simulink model "SAS_12th_question"  (R2024b)
settings: Solver=ode45  StartTime=0.0  StopTime=10.0  RelTol=1e-3
settings Model: Creator=anand  LastModifiedBy=Acer
settings RTWCC: GPUComputeCapability=3.5

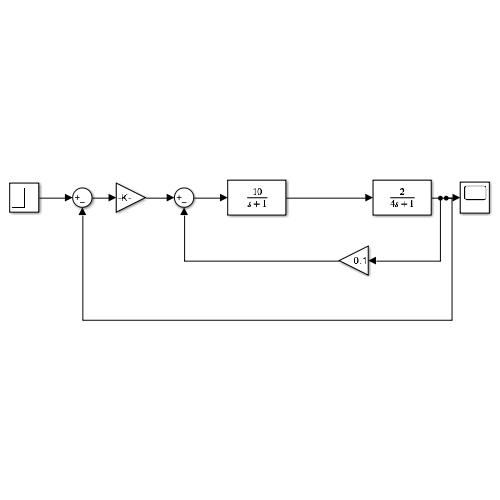
[thumbnail: Simulink's stored preview of the top-level diagram]
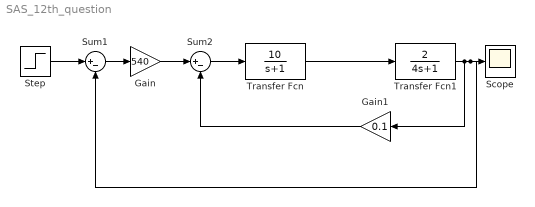
== system SAS_12th_question ==
  Gain : Gain  Gain=540
  Gain1 : Gain  Gain=0.1
  Scope : Scope
  Step : Step  SampleTime=0
  Sum1 : Sum  Inputs=|+-
  Sum2 : Sum  Inputs=|+-
  Transfer Fcn : TransferFcn  Numerator=[10]  Denominator=[1 1]
  Transfer Fcn1 : TransferFcn  Numerator=[2]  Denominator=[4 1]
  wires:
  Step/1 -> Sum1/1
  Gain/1 -> Sum2/1
  Sum2/1 -> Transfer Fcn/1
  Transfer Fcn/1 -> Transfer Fcn1/1
  Sum1/1 -> Gain/1
  Gain1/1 -> Sum2/2
  Transfer Fcn1/1 -> Gain1/1, Sum1/2, Scope/1
